simulink subsystem "SubsystemGenericDrive"  (R2020b)
settings: Solver=VariableStepAuto  StartTime=0.0  StopTime=10.0  RelTol=1e-3
settings Model: Creator=kaebi  LastModifiedBy=kaebi

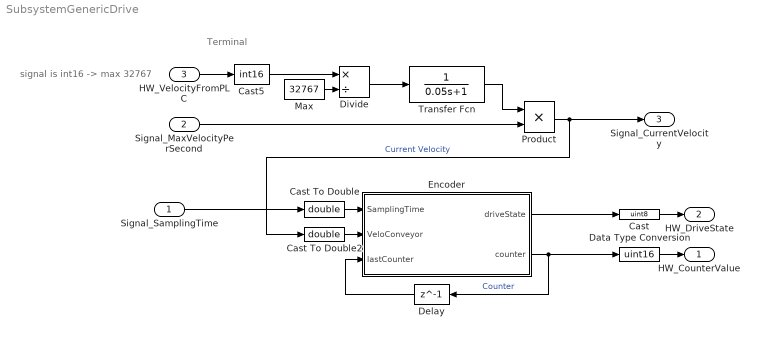
== system SubsystemGenericDrive ==
  note: signal is int16 -> max 32767
  note: Terminal
  Signal_SamplingTime : Inport
  Signal_MaxVelocityPerSecond : Inport  Port=2
  HW_VelocityFromPLC : Inport  Port=3
  Cast : DataTypeConversion  OutDataTypeStr=uint8
  Cast To Double : DataTypeConversion  OutDataTypeStr=double
  Cast To Double2 : DataTypeConversion  OutDataTypeStr=double
  Cast5 : DataTypeConversion  OutDataTypeStr=int16
  Data Type Conversion : DataTypeConversion  OutDataTypeStr=uint16  SaturateOnIntegerOverflow=on
  Delay : Delay  DelayLength=1
  Divide : Product  Inputs=*/
  Encoder : MATLAB Function  TreatAsAtomicUnit=on
  Max : Constant  Value=32767
  Product : Product
  Transfer Fcn : TransferFcn  Denominator=[0.05 1]
  HW_CounterValue : Outport
  HW_DriveState : Outport  Port=2
  Signal_CurrentVelocity : Outport  Port=3
  wires:
  Cast To Double2/1 -> Encoder/2(VeloConveyor)
  Encoder/2(counter) -> Delay/1, Data Type Conversion/1  "Counter"
  Product/1 -> Cast To Double2/1, Signal_CurrentVelocity/1  "Current Velocity"
  Data Type Conversion/1 -> HW_CounterValue/1
  Cast5/1 -> Divide/1
  Cast/1 -> HW_DriveState/1
  Delay/1 -> Encoder/3(lastCounter)
  Signal_MaxVelocityPerSecond/1 -> Product/2
  Transfer Fcn/1 -> Product/1
  Max/1 -> Divide/2
  Divide/1 -> Transfer Fcn/1
  Cast To Double/1 -> Encoder/1(SamplingTime)
  Signal_SamplingTime/1 -> Cast To Double/1
  Encoder/1(driveState) -> Cast/1
  HW_VelocityFromPLC/1 -> Cast5/1

== matlab function SubsystemGenericDrive/Encoder ==
  data: SamplingTime input; driveState output; VeloConveyor input; lastCounter input; counter output
function [driveState,counter] = GenericEncoderNew(SamplingTime, VeloConveyor, lastCounter)
%%
%    VeloConveyor in Unit/s
%    SamplingTime in s
%    lastCounter 1count = 0.0001 Unit

%%
driveState = uint8(0);
driveState = bitset(driveState,1,1);    % Ready to enable
driveState = bitset(driveState,2,1);    % Ready 
if (VeloConveyor > 0)
    driveState = bitset(driveState,5,1);    % Moving Positive
elseif (VeloConveyor < 0)
    driveState = bitset(driveState,6,1);    % Moving Negative
end

diff = VeloConveyor*SamplingTime*10000;
counter = mod(lastCounter+diff, 65535);

end
